simulink model "hvac_1zone_v3"  (R2021a)
settings: Solver=FixedStepDiscrete  StartTime=0.0  StopTime=Inf  RelTol=1e-3  EnableMultiTasking=on
values from neighbouring files (symbols this model uses):
  ci = ci'    [localResetFcn.m]
  Ts2 = 600    [main_1zone.m]
undefined symbols (not defined in the file or in its folder): den, num, params1, rl, Ts
libraries: rllib x1
settings Model: Creator=User  LastModifiedBy=Richi
settings SolverCC: AlgebraicLoopSolver=TrustRegion
settings DataIOCC: LimitDataPoints=on  SaveFormat=Array  SignalLoggingSaveFormat=ModelDataLogs
settings OptimizationCC: LifeSpan=inf
settings DebuggingCC: SolverPrmCheckMsg=warning  MultiTaskDSMMsg=warning  MultiTaskCondExecSysMsg=none  MultiTaskRateTransMsg=warning  AllowSymbolicDim=off  SFUnexpectedBacktrackingDiag=warning  SFNoUnconditionalDefaultTransitionDiag=warning  SFExecutionAtInitializationDiag=none  SFMachineParentedDataDiag=warning  ArithmeticOperatorsInVariantConditions=warning
settings HardwareCC: ProdBitPerPointer=32  ProdBitPerSizeT=32  ProdBitPerPtrDiffT=32  ProdLargestAtomicFloat=None  ProdIntDivRoundTo=Undefined  ProdEndianess=Unspecified  ProdWordSize=32  ProdHWDeviceType=32-bit Generic
settings ModelReferenceCC: PropagateSignalLabelsOutOfModel=off
settings SFSimCC: SimUseLocalCustomCode=off  CustomCodeUndefinedFunction=UseInterfaceOnly  SimTargetLang=C++
settings RTWCC: RTWUseLocalCustomCode=off
settings CodeAppCC: StateflowObjectComments=on
settings GRTTargetCC: TargetLangStandard=C89/C90 (ANSI)
settings ConfigComp: CovMetricSettings=dw  CovSaveCumulativeToWorkspaceVar=on  CovSaveSingleToWorkspaceVar=on  CovExternalEMLEnable=off

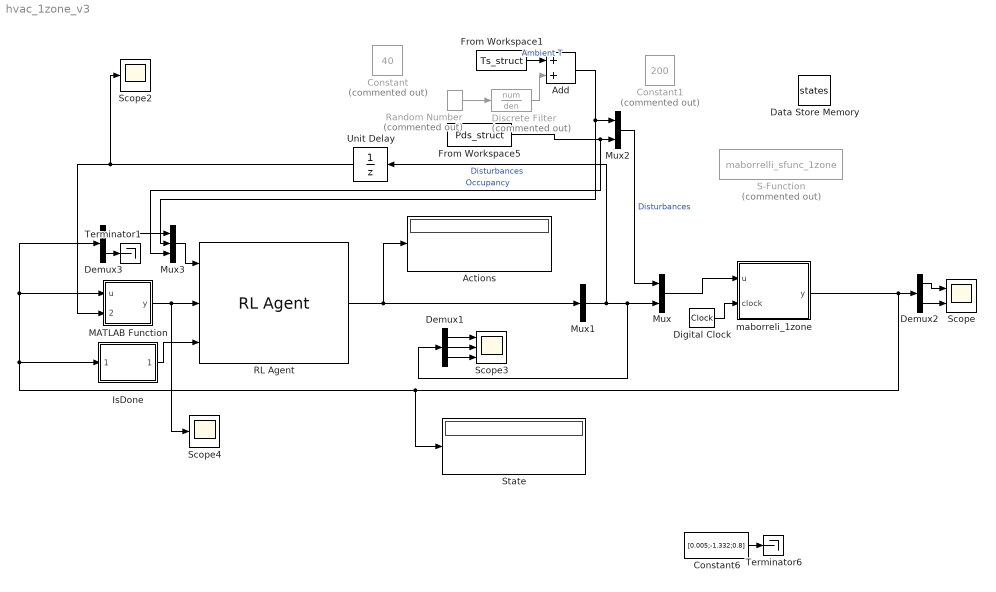
== system hvac_1zone_v3 ==
  Actions : Display
  Add : Sum
  Constant : Constant  Commented=on  Value=40
  Constant1 : Constant  Commented=on  Value=200
  Constant6 : Constant  Value=[0.005;-1.332;0.8]
  Data Store Memory : DataStoreMemory  DataStoreName=states  ReadBeforeWriteMsg=warning  WriteAfterWriteMsg=warning  WriteAfterReadMsg=warning  InitialValue=ci  VectorParams1D=off  ShowAdditionalParam=off  OutDataTypeStr=double
  Demux1 : Demux  Outputs=3
  Demux2 : Demux  Outputs=2
  Demux3 : Demux  Outputs=2
  Digital Clock : DigitalClock  SampleTime=Ts
  Discrete Filter : DiscreteFilter  Commented=on  Numerator=num  Denominator=den  SampleTime=5400
  From Workspace1 : FromWorkspace  VariableName=Ts_struct  OutDataTypeStr=double  SampleTime=-1
  From Workspace5 : FromWorkspace  VariableName=Pds_struct  OutDataTypeStr=double  SampleTime=-1
  IsDone : MATLAB Function  TreatAsAtomicUnit=on
  MATLAB Function : MATLAB Function  TreatAsAtomicUnit=on
  Mux : Mux  Inputs=2
  Mux1 : Mux  Inputs=1
  Mux2 : Mux  Inputs=2
  Mux3 : Mux  Inputs=3
  RL Agent : rllib/RL Agent  Agent=rl.util.PolicyInstance.get('hvac_1zone_v3/RL Agent')  ExternalActionAsInput=off  ProvideCumRwd=off  TreatAsDirectFeedthrough=on
  Random Number : RandomNumber  Commented=on  Variance=0.5  SampleTime=1800
  S-Function : S-Function  Commented=on  FunctionName=maborrelli_sfunc_1zone  Parameters=ci,params1,60  SFunctionDeploymentMode=off  EnableBusSupport=off
  Scope : Scope  NumInputPorts=2
  Scope2 : Scope
  Scope3 : Scope  NumInputPorts=3
  Scope4 : Scope
  State : Display
  Terminator1 : Terminator
  Terminator6 : Terminator
  Unit Delay : UnitDelay  SampleTime=Ts2  HasFrameUpgradeWarning=on
  maborreli_1zone : MATLAB Function  TreatAsAtomicUnit=on  SystemSampleTime=Ts
  wires:
  Mux2/1 -> Mux/1  "Disturbances"
  From Workspace5/1 -> Mux3/3, Mux2/2  "Occupancy"
  Mux/1 -> maborreli_1zone/1(u)
  Constant6/1 -> Terminator6/1
  Discrete Filter/1 -> Add/2
  Random Number/1 -> Discrete Filter/1
  RL Agent/1 -> Mux1/1, Actions/1
  IsDone/1(value) -> RL Agent/3
  MATLAB Function/1(y) -> Scope4/1, RL Agent/2
  maborreli_1zone/1(y) -> State/1, MATLAB Function/1(u), Demux3/1, IsDone/1(states), Demux2/1
  Demux1/2 -> Scope3/2
  Demux1/1 -> Scope3/1
  Demux1/3 -> Scope3/3
  Demux2/1 -> Scope/1
  Demux2/2 -> Scope/2
  Demux3/1 -> Mux3/1
  Demux3/2 -> Terminator1/1
  Mux1/1 -> Unit Delay/1, Demux1/1, Mux/2  "Disturbances"
  Unit Delay/1 -> Scope2/1, MATLAB Function/2(actions)
  From Workspace1/1 -> Add/1  "Ambient T"
  Mux3/1 -> RL Agent/1
  Add/1 -> Mux3/2, Mux2/1
  Digital Clock/1 -> maborreli_1zone/2(clock)

== matlab function hvac_1zone_v3/IsDone ==
  data: states input; value output
function value = fcn(states)
 low = -10;
 max = 45;
 value = 0; 
 %disp(length(block.InputPort(1).Data))
 for i=1:length(states)
     %disp(i)
     if i == 3
         break
     end
     aux = states(i);
     %disp(aux)
     if (aux < low || aux > max) 
        %disp(abs(aux - low))
        value = 1;
        break
     end
     %disp('if3')
 end

== matlab function hvac_1zone_v3/MATLAB Function ==
  data: u input; y output; actions input
function y = reward(u, actions)
 low = 22;
 high = 25;
 ms = actions(1);
 Dt = actions(2);
 %Añadir energía:
 e = ((-1012/4)*ms*Dt+ 65*(ms)^2)*2.7778e-04;
 reward = -0.8 * e; 
 %disp(length(block.InputPort(1).Data))
 for i=1:1
     %disp(i)
     aux = u(i);
     %disp(aux)
     if (aux < low || aux > high) && (abs(aux - low) >= 1 && abs(aux-high) >= 1)
        %disp(abs(aux - low))
        reward = reward - min( abs(aux - low), abs(aux - high));
        %reward = reward + 0;
        %disp('if13')
     end
     %disp('if1')
     if (aux >= low && aux <= high)
        reward = reward + 0.5;
     end

 end
y = reward;

== matlab function hvac_1zone_v3/maborreli_1zone ==
  data: u input; y output; params1 parameter; ci parameter; Ts parameter; states data_store_memory; clock input
function y = fcn(u,params1, ci, Ts, clock)
ST = Ts;
params = params1;
global states;
dT = [0;0];
delta=u(5);
if clock == 0
    dT = ci;
else
    x = states;
    dT(1)=x(1)+(ST*u(3)*params.cp*((delta*x(1)+(1-delta)*u(1)+u(4))-x(1))+ ST*(x(2)-x(1))/params.R+...
        ST*(u(1)-x(1))/params.Roa+ST*u(2))/params.C1;
    dT(2)=x(2)+ST*(x(1)-x(2))/params.R/params.C2;
end
states = dT;
y = dT;
